simulink model "apresentacao"  (R2020a)
settings: Solver=VariableStepAuto  StartTime=0.0  StopTime=2  RelTol=1e-3
values from neighbouring files (symbols this model uses):
  beta = 1/3    (= 0.333333333333)    [apresentacao_script.m]
  F = 2*sin((pi*fc)/fs)    [apresentacao_script.m]
  fs = 44100    [apresentacao_script.m]
  N = 1000    [apresentacao_script.m]
  Q = 2*0.05    (= 0.1)    [apresentacao_script.m]
  Ts = 1/44100    (= 2.26757369615e-05)    [apresentacao_script.m]
libraries: simulink x4, dspvision x2, commanapbnd3 x1
settings Model: Creator=Jose Murteira  LastModifiedBy=Jose Murteira

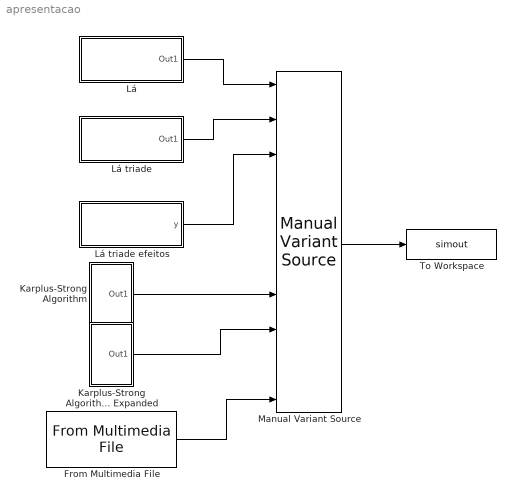
== system apresentacao ==
  From Multimedia File : dspvision/From Multimedia File  inputFilename=temp_for_effect.wav  readRange=[1 Inf]  loop=on  numPlays=inf  outputStreams=Audio only  videoDataType=single  audioDataType=double  inheritSampleTime=on  userDefinedSampleTime=1/30  noAudioOutput=off  isIntensityVideo=off  fourcc=RGB  colorVideoFormat=Separate color signals  outputEOF=off  dataOrg=Column-major  audioFrameSize=1  computeAudioFrameSize=off  outSamplingMode=Sample based
  Karplus-Strong Algorithm : Subsystem
  Karplus-Strong Algorithm Expanded : Subsystem
  Lá : Subsystem
  "Lá triade " : Subsystem
  Lá triade efeitos : Subsystem
  Manual Variant Source : simulink/Signal Routing/Manual Variant Source  NumChoices=10  LabelModeActiveChoice=V_3
  To Workspace : ToWorkspace  VariableName=simout  SaveFormat=Timeseries  SampleTime=-1
  wires:
  Lá/1(Out1) -> Manual Variant Source/1
  "Lá triade "/1(Out1) -> Manual Variant Source/2
  Lá triade efeitos/1(y) -> Manual Variant Source/3
  Karplus-Strong Algorithm/1(Out1) -> Manual Variant Source/7
  Manual Variant Source/1 -> To Workspace/1
  From Multimedia File/1 -> Manual Variant Source/10
  Karplus-Strong Algorithm Expanded/1(Out1) -> Manual Variant Source/8

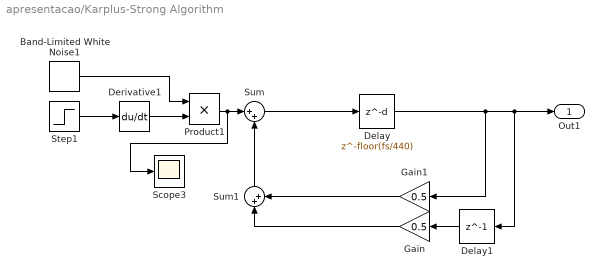
== system apresentacao/Karplus-Strong Algorithm ==
  Band-Limited White Noise1 : simulink/Sources/Band-Limited White Noise  Cov=[0.01]  Ts=Ts  seed=[23341]
  Delay : Delay  DelayLength=floor(fs/440)  InitialCondition=0  SampleTime=Ts
  Delay1 : Delay  DelayLength=1  InitialCondition=0
  Derivative1 : Derivative
  Gain : Gain  Gain=0.5
  Gain1 : Gain  Gain=0.5
  Product1 : Product
  Scope3 : Scope
  Step1 : Step  Time=0.01  SampleTime=1/44000
  Sum : Sum  Inputs=|++
  Sum1 : Sum  Inputs=|++
  Out1 : Outport
  wires:
  Product1/1 -> Scope3/1, Sum/1
  Step1/1 -> Derivative1/1
  Derivative1/1 -> Product1/2
  Gain1/1 -> Sum1/2
  Band-Limited White Noise1/1 -> Product1/1
  Sum/1 -> Delay/1
  Sum1/1 -> Sum/2
  Gain/1 -> Sum1/1
  Delay1/1 -> Gain/1
  Delay/1 -> Gain1/1, Out1/1, Delay1/1

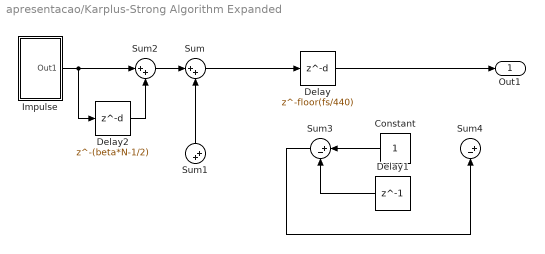
== system apresentacao/Karplus-Strong Algorithm Expanded ==
  Constant : Constant
  Delay : Delay  DelayLength=floor(fs/440)  InitialCondition=0  SampleTime=Ts
  Delay1 : Delay  DelayLength=1  InitialCondition=0
  Delay2 : Delay  DelayLength=(beta*N-1/2)  InitialCondition=0
  Impulse : Subsystem
  Sum : Sum  Inputs=|++
  Sum1 : Sum  Inputs=|++
  Sum2 : Sum  Inputs=|++
  Sum3 : Sum  Inputs=|+-
  Sum4 : Sum  Inputs=|+-
  Out1 : Outport
  wires:
  Sum/1 -> Delay/1
  Sum1/1 -> Sum/2
  Delay/1 -> Out1/1
  Sum2/1 -> Sum/1
  Delay2/1 -> Sum2/2
  Impulse/1(Out1) -> Sum2/1, Delay2/1
  Constant/1 -> Sum3/1
  Delay1/1 -> Sum3/2
  Sum3/1 -> Sum4/2

== system apresentacao/Lá ==
  Sine Wave : Sin  Frequency=440*pi*2  SampleTime=Ts
  Out1 : Outport
  wires:
  Sine Wave/1 -> Out1/1

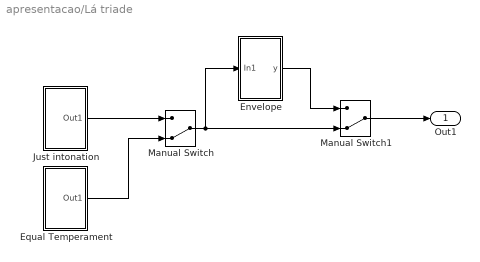
== system apresentacao/Lá triade  ==
  Envelope : Subsystem
  Equal Temperament : Subsystem
  Just intonation : Subsystem
  Manual Switch : ManualSwitch  CurrentSetting=0
  Manual Switch1 : ManualSwitch  CurrentSetting=0
  Out1 : Outport
  wires:
  Just intonation/1(Out1) -> Manual Switch/1
  Equal Temperament/1(Out1) -> Manual Switch/2
  Manual Switch/1 -> Envelope/1(In1), Manual Switch1/2
  Manual Switch1/1 -> Out1/1
  Envelope/1(y) -> Manual Switch1/1

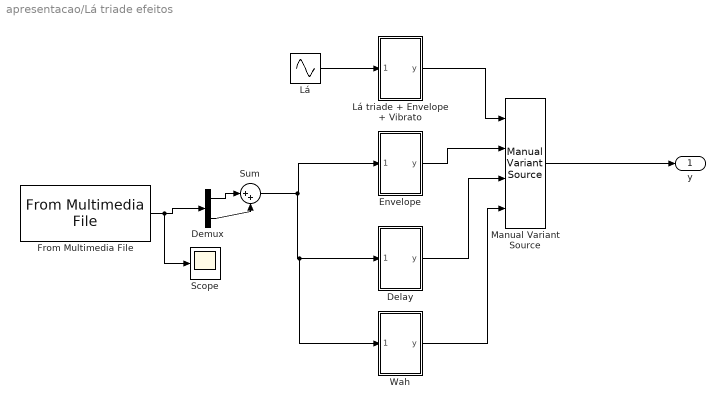
== system apresentacao/Lá triade efeitos ==
  " Wah" : Subsystem
  "Delay " : Subsystem
  Demux : Demux  Outputs=2
  "Envelope " : Subsystem
  From Multimedia File : dspvision/From Multimedia File  inputFilename=temp_for_effect.wav  readRange=[1 Inf]  loop=on  numPlays=inf  outputStreams=Audio only  videoDataType=single  audioDataType=double  inheritSampleTime=on  userDefinedSampleTime=1/30  noAudioOutput=off  isIntensityVideo=off  fourcc=RGB  colorVideoFormat=Separate color signals  outputEOF=off  dataOrg=Column-major  audioFrameSize=1  computeAudioFrameSize=off  outSamplingMode=Sample based
  Lá : Sin  Frequency=440*pi*2  SampleTime=Ts
  Lá triade + Envelope + Vibrato : Subsystem
  Manual Variant Source : simulink/Signal Routing/Manual Variant Source  NumChoices=4  LabelModeActiveChoice=V_4
  Scope : Scope
  Sum : Sum  Inputs=|++
  y : Outport
  wires:
  Lá triade + Envelope + Vibrato/1(y) -> Manual Variant Source/1
  "Envelope "/1(y) -> Manual Variant Source/2
  "Delay "/1(y) -> Manual Variant Source/3
  " Wah"/1(y) -> Manual Variant Source/4
  From Multimedia File/1 -> Scope/1, Demux/1
  Demux/1 -> Sum/1
  Demux/2 -> Sum/2
  Manual Variant Source/1 -> y/1
  Lá/1 -> Lá triade + Envelope + Vibrato/1(Input)
  Sum/1 -> " Wah"/1(Input), "Delay "/1(Input), "Envelope "/1(Input)

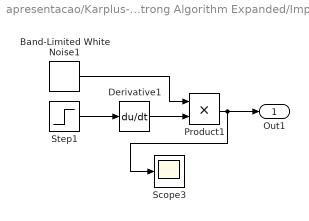
== system apresentacao/Karplus-Strong Algorithm Expanded/Impulse ==
  Band-Limited White Noise1 : simulink/Sources/Band-Limited White Noise  Cov=[0.01]  Ts=Ts  seed=[23341]
  Derivative1 : Derivative
  Product1 : Product
  Scope3 : Scope
  Step1 : Step  Time=0.01  SampleTime=1/44000
  Out1 : Outport
  wires:
  Derivative1/1 -> Product1/2
  Band-Limited White Noise1/1 -> Product1/1
  Step1/1 -> Derivative1/1
  Product1/1 -> Out1/1, Scope3/1

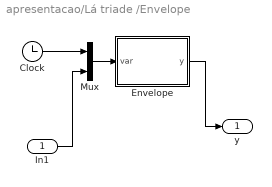
== system apresentacao/Lá triade /Envelope ==
  In1 : Inport
  Clock : Clock
  Envelope : MATLAB Function  TreatAsAtomicUnit=on
  Mux : Mux  Inputs=2
  y : Outport
  wires:
  Clock/1 -> Mux/1
  In1/1 -> Mux/2
  Envelope/1(y) -> y/1
  Mux/1 -> Envelope/1(var)

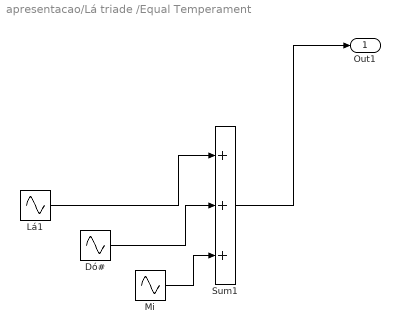
== system apresentacao/Lá triade /Equal Temperament ==
  Dó# : Sin  Frequency=440*pi*2*(2^(4/12))  SampleTime=Ts
  Lá1 : Sin  Frequency=440*pi*2  SampleTime=Ts
  Mi : Sin  Frequency=440*pi*2*(2^(7/12))  SampleTime=Ts
  Sum1 : Sum  Inputs=|+++
  Out1 : Outport
  wires:
  Mi/1 -> Sum1/3
  Lá1/1 -> Sum1/1
  Dó#/1 -> Sum1/2
  Sum1/1 -> Out1/1

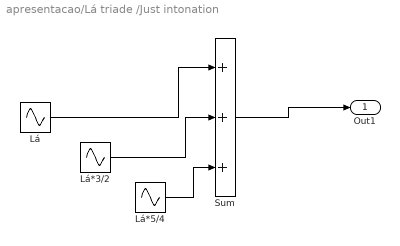
== system apresentacao/Lá triade /Just intonation ==
  Lá : Sin  Frequency=440*pi*2  SampleTime=Ts
  Lá*3/2 : Sin  Frequency=440*pi*2*3/2  SampleTime=Ts
  Lá*5/4 : Sin  Frequency=440*pi*2*5/4  SampleTime=Ts
  Sum : Sum  Inputs=|+++
  Out1 : Outport
  wires:
  Sum/1 -> Out1/1
  Lá/1 -> Sum/1
  Lá*3/2/1 -> Sum/2
  Lá*5/4/1 -> Sum/3

== system apresentacao/Lá triade efeitos/ Wah ==
  Input : Inport
  Scope : Scope
  Wah : Subsystem
  y : Outport
  wires:
  Input/1 -> Wah/1(Input)
  Wah/1(y) -> y/1, Scope/1

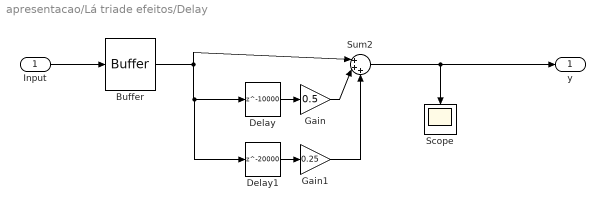
== system apresentacao/Lá triade efeitos/Delay  ==
  Input : Inport
  Buffer : Buffer  N=1  OutputFrames=off
  Delay : Delay  DelayLength=10000
  Delay1 : Delay  DelayLength=20000
  Gain : Gain  Gain=0.5
  Gain1 : Gain  Gain=0.25
  Scope : Scope
  Sum2 : Sum  Inputs=|+++
  y : Outport
  wires:
  Sum2/1 -> y/1, Scope/1
  Delay1/1 -> Gain1/1
  Delay/1 -> Gain/1
  Buffer/1 -> Delay1/1, Delay/1, Sum2/1
  Input/1 -> Buffer/1
  Gain/1 -> Sum2/2
  Gain1/1 -> Sum2/3

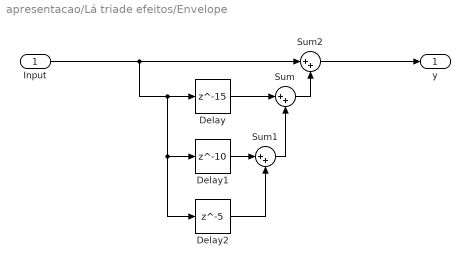
== system apresentacao/Lá triade efeitos/Envelope  ==
  Input : Inport
  Delay : Delay  DelayLength=15
  Delay1 : Delay  DelayLength=10
  Delay2 : Delay  DelayLength=5
  Sum : Sum  Inputs=|++
  Sum1 : Sum  Inputs=|++
  Sum2 : Sum  Inputs=|++
  y : Outport
  wires:
  Sum2/1 -> y/1
  Delay/1 -> Sum/1
  Sum1/1 -> Sum/2
  Delay1/1 -> Sum1/1
  Delay2/1 -> Sum1/2
  Input/1 -> Delay2/1, Delay1/1, Delay/1, Sum2/1
  Sum/1 -> Sum2/2

== system apresentacao/Lá triade efeitos/Lá triade + Envelope + Vibrato ==
  Input : Inport
  FM Modulator Passband : commanapbnd3/FM Modulator Passband  Fc=440  Ph=pi/2  Kc=5000
      settings: SourceProductBaseCode=CM
  y : Outport
  wires:
  Input/1 -> FM Modulator Passband/1
  FM Modulator Passband/1 -> y/1

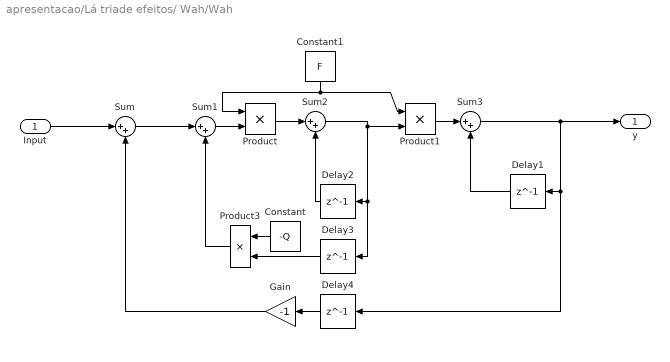
== system apresentacao/Lá triade efeitos/ Wah/Wah ==
  Input : Inport
  Constant : Constant  Value=-Q
  Constant1 : Constant  Value=F
  Delay{1..4} (4 alike) : Delay  DelayLength=1  InitialCondition=0
  Gain : Gain  Gain=-1
  Product : Product
  Product1 : Product
  Product3 : Product
  Sum{,1..3} (4 alike) : Sum  Inputs=|++
  y : Outport
  wires:
  Constant1/1 -> Product/1, Product1/1
  Product/1 -> Sum2/1
  Gain/1 -> Sum/2
  Delay2/1 -> Sum2/2
  Product1/1 -> Sum3/1
  Constant/1 -> Product3/1
  Sum3/1 -> y/1, Delay4/1, Delay1/1
  Sum/1 -> Sum1/1
  Input/1 -> Sum/1
  Sum1/1 -> Product/2
  Sum2/1 -> Product1/2, Delay3/1, Delay2/1
  Product3/1 -> Sum1/2
  Delay1/1 -> Sum3/2
  Delay3/1 -> Product3/2
  Delay4/1 -> Gain/1

== matlab function apresentacao/Lá triade /Envelope/Envelope ==
  data: var input; y output
function y = fcn(var)
t=var(1);
if(t<0.003)
    g=0.1/0.03*t;
else
   g=1.8^(-(t-0.03));
end
y = var(2)*(g);
